simulink model "systemFSM"  (R2022b)
settings: Solver=FixedStepDiscrete  StartTime=0.0  StopTime=20  FixedStep=0.01  RelTol=1e-3  EnableMultiTasking=on
settings Model: Creator=RJRose  LastModifiedBy=RJRose
settings SolverCC: AlgebraicLoopSolver=TrustRegion  AutoInsertRateTranBlk=on
settings DataIOCC: LimitDataPoints=on
settings OptimizationCC: LifeSpan=inf
settings DebuggingCC: UnconnectedInputMsg=warning  UnconnectedOutputMsg=warning  UnconnectedLineMsg=warning  AllowSymbolicDim=off  SFUnexpectedBacktrackingDiag=warning  SFNoUnconditionalDefaultTransitionDiag=warning  SFExecutionAtInitializationDiag=none  ArithmeticOperatorsInVariantConditions=warning
settings ModelReferenceCC: EnableRefExpFcnMdlSchedulingChecks=on
settings SFSimCC: SimUseLocalCustomCode=off  CustomCodeUndefinedFunction=UseInterfaceOnly
settings RTWCC: RTWUseLocalCustomCode=off  DLArmComputeVersion=19.05
settings CodeAppCC: StateflowObjectComments=on
settings GRTTargetCC: TargetLangStandard=C89/C90 (ANSI)
settings ConfigComp: CovMetricSettings=dw  CovSaveCumulativeToWorkspaceVar=on  CovSaveSingleToWorkspaceVar=on  CovExternalEMLEnable=off  CovSFcnEnable=off

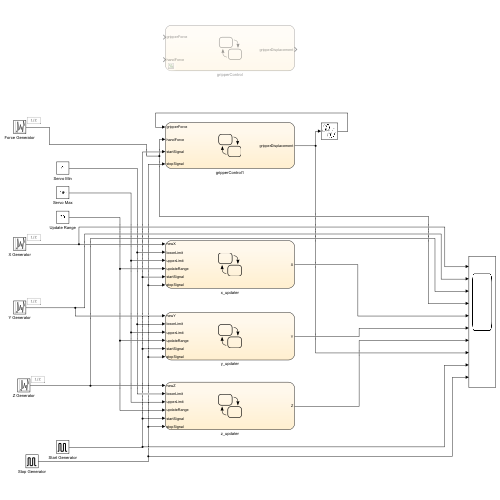
[thumbnail: Simulink's stored preview of the top-level diagram]
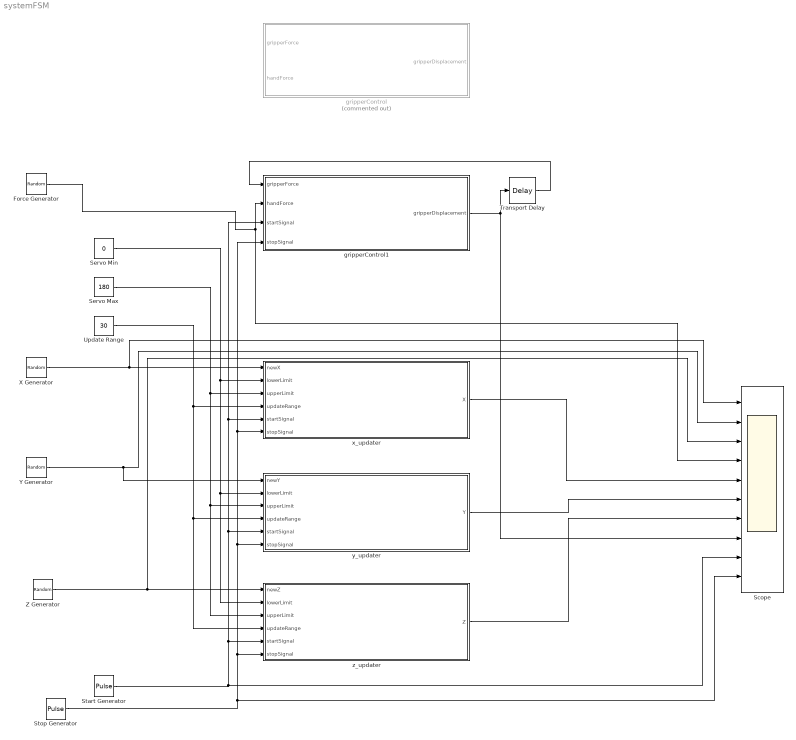
== system systemFSM ==
  Force Generator : UniformRandomNumber  Minimum=1  Maximum=71  Seed=4  SampleTime=0.1
  Scope : Scope  NumInputPorts=10
  Servo Max : Constant  Value=180
  Servo Min : Constant  Value=0
  Start Generator : DiscretePulseGenerator  PulseType=Time based  Period=20  PulseWidth=5  PhaseDelay=5
  Stop Generator : DiscretePulseGenerator  PulseType=Time based  Period=20  PulseWidth=5  PhaseDelay=15
  Transport Delay : TransportDelay  DelayTime=.5
  Update Range : Constant  Value=30
  X Generator : UniformRandomNumber  Minimum=0  Maximum=360  SampleTime=0.1
  Y Generator : UniformRandomNumber  Minimum=0  Maximum=180  Seed=1  SampleTime=0.1
  Z Generator : UniformRandomNumber  Minimum=0  Maximum=180  Seed=2  SampleTime=0.1
  gripperControl : Stateflow chart  Commented=on  TreatAsAtomicUnit=on
  gripperControl1 : Stateflow chart  TreatAsAtomicUnit=on
  x_updater : Stateflow chart  TreatAsAtomicUnit=on
  y_updater : Stateflow chart  TreatAsAtomicUnit=on
  z_updater : Stateflow chart  TreatAsAtomicUnit=on
  wires:
  Servo Min/1 -> z_updater/2(lowerLimit), y_updater/2(lowerLimit), x_updater/2(lowerLimit)
  Servo Max/1 -> z_updater/3(upperLimit), y_updater/3(upperLimit), x_updater/3(upperLimit)
  Update Range/1 -> z_updater/4(updateRange), y_updater/4(updateRange), x_updater/4(updateRange)
  Z Generator/1 -> z_updater/1(newZ), Scope/3
  X Generator/1 -> Scope/1, x_updater/1(newX)
  Y Generator/1 -> y_updater/1(newY), Scope/2
  x_updater/1(X) -> Scope/5
  y_updater/1(Y) -> Scope/6
  z_updater/1(Z) -> Scope/7
  Force Generator/1 -> Scope/4, gripperControl1/2(handForce)
  gripperControl1/1(gripperDisplacement) -> Transport Delay/1, Scope/8
  Transport Delay/1 -> gripperControl1/1(gripperForce)
  Start Generator/1 -> gripperControl1/3(startSignal), x_updater/5(startSignal), y_updater/5(startSignal), z_updater/5(startSignal), Scope/9
  Stop Generator/1 -> gripperControl1/4(stopSignal), x_updater/6(stopSignal), y_updater/6(stopSignal), z_updater/6(stopSignal), Scope/10

== stateflow chart systemFSM/gripperControl1 ==
  state Active
  state Stopped
  Active -> Active [order 2] : [handForce < 10 && gripperDisplacement>GDmin]
      | {gripperDisplacement = gripperDisplacement - 10}
  Active -> Active [order 1] : [handForce - gripperForce > 10 && gripperDisplacement<GDmax]
      | {gripperDisplacement = gripperDisplacement + 5}
  Stopped -> Active : [startSignal == 1]
  Active -> Stopped [order 3] : [stopSignal == 1]
  (default) -> Stopped : {gripperDisplacement = 10}
  data: gripperForce input; handForce input; GDmin constant double =10; gripperDisplacement output; GDmax constant double =71; startSignal input; stopSignal input

== stateflow chart systemFSM/y_updater ==
  state Active
  state Stopped
  Active -> Active [order 1] : [(newY<Y+updateRange&&newY>Y-updateRange)&&(newY<=upperLimit)&&(newY>=lowerLimit)]{Y = newY}
  Active -> Stopped [order 2] : [stopSignal == 1]
  Stopped -> Active : [startSignal == 1]
  (default) -> Stopped : {Y = 90}
  data: newY input; Y output; lowerLimit input; upperLimit input; updateRange input; startSignal input; stopSignal input

== stateflow chart systemFSM/gripperControl ==
  state Gripping
  state Idle
  state Releasing
  Gripping -> Idle [order 1] : [handForce<=gripperForce||gripperDisplacement>=GDmax]
  Releasing -> Idle [order 1] : [handForce>=gripperForce||gripperDisplacement<=GDmin]
  Idle -> Idle [order 1] : [handForce==gripperForce]
  (default) -> Idle
  Gripping -> Gripping [order 2] : [handForce>gripperForce&&gripperDisplacement<GDmax]
      | {gripperDisplacement == gripperDisplacement + 1}
  Releasing -> Releasing [order 2] : [handForce<gripperForce&&gripperDisplacement>GDmin]
      | {gripperDisplacement == gripperDisplacement - 1}
  Idle -> Gripping [order 3] : [handForce>gripperForce]
  Idle -> Releasing [order 2] : [handForce<gripperForce]
  data: gripperForce input; handForce input; GDmin constant double =10; gripperDisplacement output; GDmax constant double =71

== stateflow chart systemFSM/z_updater ==
  state Active
  state Stopped
  Active -> Active [order 1] : [(newZ<Z+updateRange&&newZ>Z-updateRange)&&(newZ<=upperLimit)&&(newZ>=lowerLimit)]{Z = newZ}
  Active -> Stopped [order 2] : [stopSignal == 1]
  Stopped -> Active : [startSignal == 1]
  (default) -> Stopped : {Z = 90}
  data: newZ input; Z output; lowerLimit input; upperLimit input; updateRange input; startSignal input; stopSignal input

== stateflow chart systemFSM/x_updater ==
  state Active
  state Stopped
  Active -> Active [order 1] : [(newX<X+updateRange&&newX>X-updateRange)&&(newX<=upperLimit)&&(newX>=lowerLimit)]{X = newX}
  Active -> Stopped [order 2] : [stopSignal == 1]
  Stopped -> Active : [startSignal == 1]
  (default) -> Stopped : {X = 90}
  data: newX input; X output; lowerLimit input; upperLimit input; updateRange input; startSignal input; stopSignal input
